simulink model "temp_simulink"  (R2024a)
settings: Solver=ode4  StartTime=0.0  StopTime=10.0  FixedStep=0.1  RelTol=1e-3
values from neighbouring files (symbols this model uses):
  A = [0, 1 ,0 ,0 ; (M+m)*g/(M*l), 0, 0, 0; 0, 0, 0, 1; -m*g/M, 0, 0, 0 ]    [temp.m]
  B = [0; -1/(M*l); 0; 1/M]    [temp.m]
  K = Kc(1:4)    [temp.m]
  Ki = -Kc(5)    [temp.m]
settings Model: Creator=caugu  LastModifiedBy=caugu

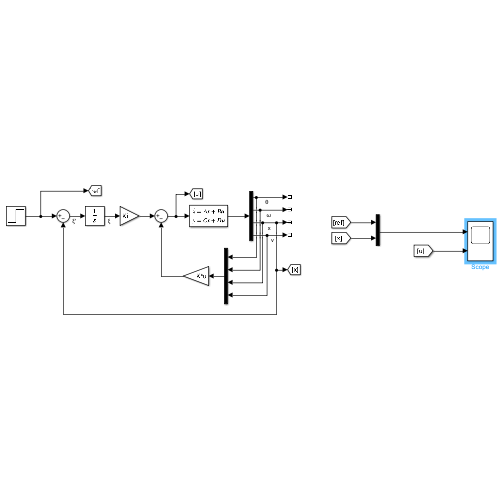
[thumbnail: Simulink's stored preview of the top-level diagram]
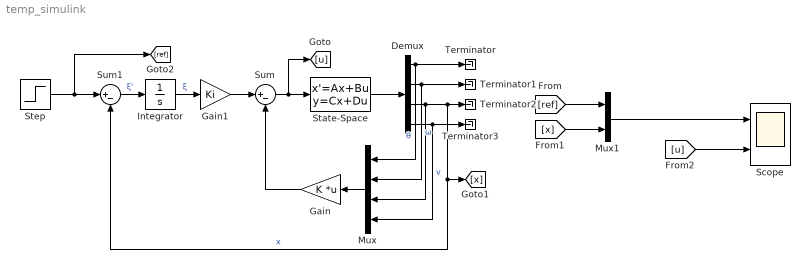
== system temp_simulink ==
  Demux : Demux
  Gain : Gain  Gain=K  Multiplication=Matrix(K*u)
  Gain1 : Gain  Gain=Ki
  Integrator : Integrator
  Mux : Mux
  Mux1 : Mux  Inputs=2
  Scope : Scope  NumInputPorts=2
  State-Space : StateSpace  A=A  B=B  C=eye(4)  D=zeros(4,1)  InitialCondition=0
  Step : Step  Time=3  SampleTime=0
  Sum : Sum  Inputs=|+-
  Sum1 : Sum  Inputs=|+-
  Terminator{,1..3} (4 alike) : Terminator
  wires:
  Demux/1 -> Mux/1, Terminator/1  "θ"
  Demux/2 -> Mux/2, Terminator1/1  "ω"
  Demux/3 -> Mux/3, [x], Sum1/2, Terminator2/1  "x"
  Demux/4 -> Mux/4, Terminator3/1  "v"
  State-Space/1 -> Demux/1
  Mux/1 -> Gain/1
  Gain/1 -> Sum/2
  Sum/1 -> [u], State-Space/1
  Gain1/1 -> Sum/1
  Integrator/1 -> Gain1/1  "ξ"
  Sum1/1 -> Integrator/1  "ξ'"
  Step/1 -> [ref], Sum1/1
  Mux1/1 -> Scope/1
  [ref] -> Mux1/1
  [x] -> Mux1/2
  [u] -> Scope/2
